simulink model "bldc_motor_sim_v2"  (R2024b)
settings: Solver=VariableStepAuto  StartTime=0.0  StopTime=1  RelTol=1e-3
undefined symbols (not defined in the file): closed_loop, D_m, DiscIntNeverNeededParam, J_t, L_ss, lambda_m, P, r_s, R_vs, V_bus
libraries: spsMosfetLib x6, spsSeriesRLCBranchLib x4, spsVoltageMeasurementLib x3, spsControlledCurrentSourceLib x3, embmathops x1, spsPWMGeneratorDCDCLib x1, spsDCVoltageSourceLib x1, sps_lib x1
settings Model: Creator=Aether  LastModifiedBy=Aether

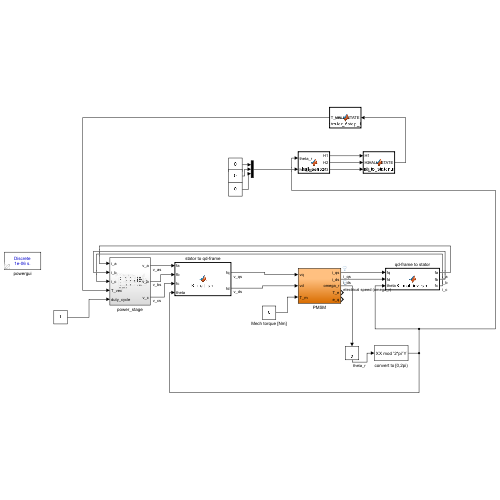
[thumbnail: Simulink's stored preview of the top-level diagram]
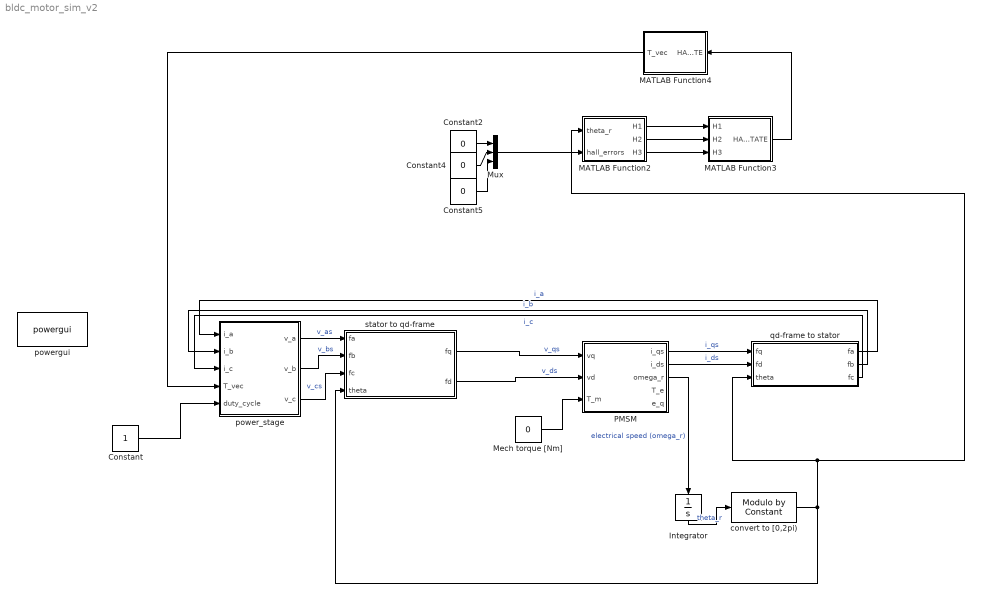
== system bldc_motor_sim_v2 ==
  Constant : Constant
  Constant2 : Constant  Value=0
  Constant4 : Constant  Value=0
  Constant5 : Constant  Value=0
  Integrator : Integrator
  MATLAB Function2 : MATLAB Function  TreatAsAtomicUnit=on
  MATLAB Function3 : MATLAB Function  TreatAsAtomicUnit=on
  MATLAB Function4 : MATLAB Function  TreatAsAtomicUnit=on
  Mech torque [Nm] : Constant  Value=0
  Mux : Mux  Inputs=3
  PMSM : Subsystem
  convert to [0,2pi) : embmathops/Modulo by Constant  Denominator=2*pi  SimulateUsing=Code generation
      settings: LibrarySourceBlock=embeddedMathLib/Modulo by Constant
  power_stage : Subsystem
  powergui : sps_lib/powergui  Priority=1  SimulationMode=Discrete  SampleTime=1e-6  frequency=60  Iterations=50  frequencyindice=0  Pbase=100e6  ErrMax=1e-4  UnitsV=kV  UnitsW=MW  buscounter=0  FunctionMessages=off  echomessages=off  EnableUseOfTLC=off  CurrentSourceSwitches=off  DisableSnubberDevices=off  DisableRonSwitches=off  DisableVfSwitches=off  DisplayEquations=off  AutomaticDiscreteSolvers=off  SolverType=Tustin/Backward Euler (TBE)  Interpol=off  ExternalGateDelay=off  methode=off  Ts=100  x0status=blocks  SPID=on  SwTol=0  HookPort=off  NonlinearTolerance=1e-4  nMaxIteration=100  ContinueOnMaxIteration=off  RestoreLinks=warning  ResistiveCurrentMeasurement=off  Frange=[0:2:500]  Ylog=off  Xlog=on  ShowGrid=off  save=off  variable=ZData  structure=0  ZoomFFT=off  StartTime=0.0  cycles=1  DisplayStyle=1  fundamental=60  FreqAxis=off  MaxFrequency=1000  frequencyindicesteady=1  RmsSteady=1  display=off
  qd-frame to stator : MATLAB Function  TreatAsAtomicUnit=on
  stator to qd-frame : MATLAB Function  TreatAsAtomicUnit=on
  wires:
  MATLAB Function4/1(T_vec) -> power_stage/4(T_vec)
  MATLAB Function2/2(H2) -> MATLAB Function3/2(H2)
  MATLAB Function2/3(H3) -> MATLAB Function3/3(H3)
  MATLAB Function3/1(HALL_STATE) -> MATLAB Function4/1(HALL_STATE)
  MATLAB Function2/1(H1) -> MATLAB Function3/1(H1)
  power_stage/1(v_a) -> stator to qd-frame/1(fa)  "v_as"
  power_stage/2(v_b) -> stator to qd-frame/2(fb)  "v_bs"
  power_stage/3(v_c) -> stator to qd-frame/3(fc)  "v_cs"
  stator to qd-frame/1(fq) -> PMSM/1(vq)  "v_qs"
  stator to qd-frame/2(fd) -> PMSM/2(vd)  "v_ds"
  Mech torque [Nm]/1 -> PMSM/3(T_m)
  PMSM/1(i_qs) -> qd-frame to stator/1(fq)  "i_qs"
  PMSM/2(i_ds) -> qd-frame to stator/2(fd)  "i_ds"
  Integrator/1 -> convert to [0,2pi)/1  "theta_r"
  PMSM/3(omega_r) -> Integrator/1  "electrical speed (omega_r)"
  convert to [0,2pi)/1 -> MATLAB Function2/1(theta_r), qd-frame to stator/3(theta), stator to qd-frame/4(theta)
  qd-frame to stator/1(fa) -> power_stage/1(i_a)  "i_a"
  qd-frame to stator/2(fb) -> power_stage/2(i_b)  "i_b"
  qd-frame to stator/3(fc) -> power_stage/3(i_c)  "i_c"
  Constant/1 -> power_stage/5(duty_cycle)
  Constant2/1 -> Mux/1
  Constant5/1 -> Mux/3
  Mux/1 -> MATLAB Function2/2(hall_errors)
  Constant4/1 -> Mux/2

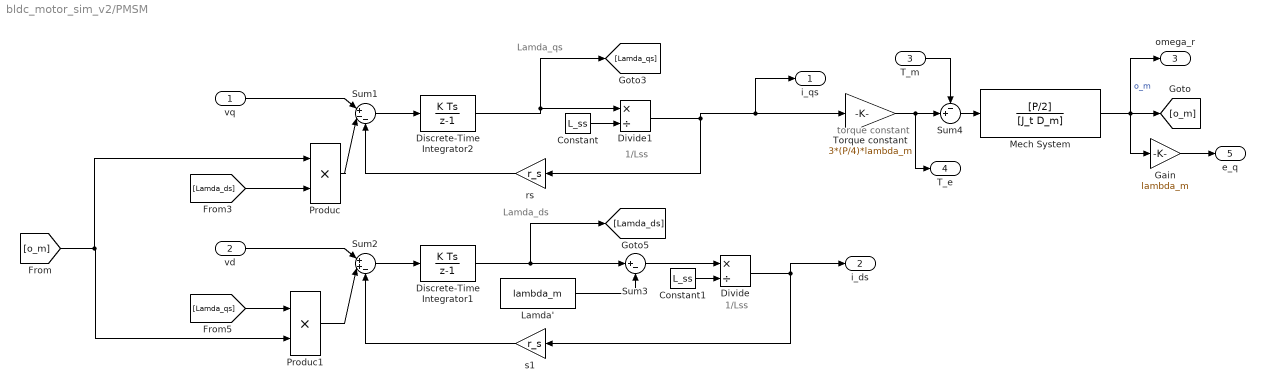
== system bldc_motor_sim_v2/PMSM ==
  note: torque constant
  note: Lamda_ds
  note: Lamda_qs
  note: 1/Lss
  note: 1/Lss
  vq : Inport
  vd : Inport  Port=2
  T_m : Inport  Port=3
  Constant : Constant  Value=L_ss
  Constant1 : Constant  Value=L_ss
  Discrete-Time Integrator1 : DiscreteIntegrator  SampleTime=-1  ICPrevOutput=DiscIntNeverNeededParam  ICPrevScaledInput=DiscIntNeverNeededParam
  Discrete-Time Integrator2 : DiscreteIntegrator  SampleTime=-1  ICPrevOutput=DiscIntNeverNeededParam  ICPrevScaledInput=DiscIntNeverNeededParam
  Divide : Product  Inputs=*/
  Divide1 : Product  Inputs=*/
  Gain : Gain  Gain=lambda_m
  Lamda' : Constant  Value=lambda_m
  Mech System : TransferFcn  Numerator=[P/2]  Denominator=[J_t D_m]
  Produc : Product  RndMeth=Zero
  Produc1 : Product  RndMeth=Zero
  Sum1 : Sum  Inputs=|+--
  Sum2 : Sum  Inputs=|++-
  Sum3 : Sum  Inputs=|+-
  Sum4 : Sum  Inputs=-+|
  Torque constant : Gain  Gain=3*(P/4)*lambda_m
  rs : Gain  Gain=r_s
  s1 : Gain  Gain=r_s
  i_qs : Outport
  i_ds : Outport  Port=2
  omega_r : Outport  Port=3
  T_e : Outport  Port=4
  e_q : Outport  Port=5
  wires:
  vd/1 -> Sum2/1
  vq/1 -> Sum1/1
  [Lamda_qs] -> Produc1/1
  [Lamda_ds] -> Produc/2
  [o_m] -> Produc1/2, Produc/1
  Lamda'/1 -> Sum3/2
  Sum3/1 -> Divide/1
  s1/1 -> Sum2/3
  Discrete-Time Integrator1/1 -> [Lamda_ds], Sum3/1
  Sum2/1 -> Discrete-Time Integrator1/1
  Produc1/1 -> Sum2/2
  Divide1/1 -> i_qs/1, Torque constant/1, rs/1
  rs/1 -> Sum1/3
  Discrete-Time Integrator2/1 -> [Lamda_qs], Divide1/1
  Sum1/1 -> Discrete-Time Integrator2/1
  Produc/1 -> Sum1/2
  Torque constant/1 -> Sum4/2, T_e/1
  Divide/1 -> i_ds/1, s1/1
  T_m/1 -> Sum4/1
  Sum4/1 -> Mech System/1
  Constant/1 -> Divide1/2
  Constant1/1 -> Divide/2
  Mech System/1 -> Gain/1, omega_r/1, [o_m]  "o_m"
  Gain/1 -> e_q/1

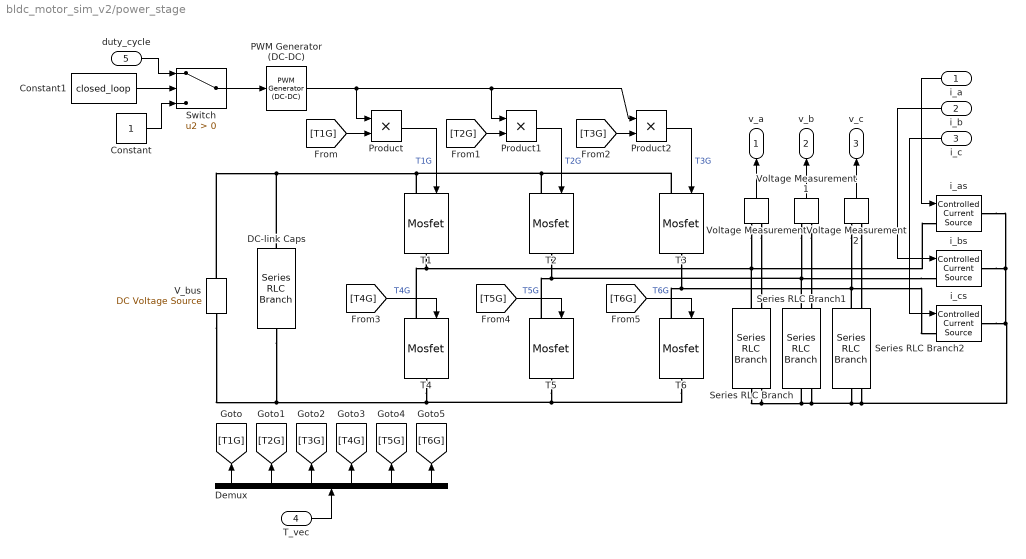
== system bldc_motor_sim_v2/power_stage ==
  i_a : Inport
  i_b : Inport  Port=2
  i_c : Inport  Port=3
  T_vec : Inport  Port=4
  duty_cycle : Inport  Port=5
  Constant : Constant
  Constant1 : Constant  Value=closed_loop
  DC-link Caps : spsSeriesRLCBranchLib/Series RLC Branch  LConnTagsString=__new0  RConnTagsString=__new0  BranchType=RC  Resistance=1e-6  Inductance=0  SetiL0=off  InitialCurrent=0  Capacitance=100e-6  Setx0=off  InitialVoltage=0  Measurements=None
  Demux : Demux  Outputs=6
  PWM Generator (DC-DC) : spsPWMGeneratorDCDCLib/PWM Generator (DC-DC)  Fsw=f_SW_Hz  Ts=0
  Product : Product
  Product1 : Product
  Product2 : Product
  Series RLC Branch : spsSeriesRLCBranchLib/Series RLC Branch  LConnTagsString=__new0  RConnTagsString=__new0  BranchType=R  Resistance=R_vs  Inductance=0  SetiL0=off  InitialCurrent=0  Capacitance=inf  Setx0=off  InitialVoltage=0  Measurements=None
  Series RLC Branch1 : spsSeriesRLCBranchLib/Series RLC Branch  LConnTagsString=__new0  RConnTagsString=__new0  BranchType=R  Resistance=R_vs  Inductance=0  SetiL0=off  InitialCurrent=0  Capacitance=inf  Setx0=off  InitialVoltage=0  Measurements=None
  Series RLC Branch2 : spsSeriesRLCBranchLib/Series RLC Branch  LConnTagsString=__new0  RConnTagsString=__new0  BranchType=R  Resistance=R_vs  Inductance=0  SetiL0=off  InitialCurrent=0  Capacitance=inf  Setx0=off  InitialVoltage=0  Measurements=None
  Switch : Switch  Criteria=u2 > Threshold  SaturateOnIntegerOverflow=off  InputSameDT=off
  T{1..6} (6 alike) : spsMosfetLib/Mosfet  Ron=R_dsON_Ohm  Lon=0  Rd=0.01  Vfd=0.7  IC=0  Rs=1e5  Cs=inf  Measurements=off
  V_bus : spsDCVoltageSourceLib/DC Voltage Source  Amplitude=V_bus  Measurements=None
  Voltage Measurement : spsVoltageMeasurementLib/Voltage Measurement  PhasorSimulation=off  OutputType=Complex  PSBequivalent=0
  Voltage Measurement1 : spsVoltageMeasurementLib/Voltage Measurement  PhasorSimulation=off  OutputType=Complex  PSBequivalent=0
  Voltage Measurement2 : spsVoltageMeasurementLib/Voltage Measurement  PhasorSimulation=off  OutputType=Complex  PSBequivalent=0
  i_as : spsControlledCurrentSourceLib/Controlled Current Source  Initialize=on  Source_Type=AC  Amplitude=0  Phase=0  Frequency=0  Measurements=None
  i_bs : spsControlledCurrentSourceLib/Controlled Current Source  Initialize=on  Source_Type=AC  Amplitude=0  Phase=0  Frequency=0  Measurements=None
  i_cs : spsControlledCurrentSourceLib/Controlled Current Source  Initialize=on  Source_Type=AC  Amplitude=0  Phase=0  Frequency=0  Measurements=None
  v_a : Outport
  v_b : Outport  Port=2
  v_c : Outport  Port=3
  wires:
  T_vec/1 -> Demux/1
  Product1/1 -> T2/1  "T2G"
  PWM Generator (DC-DC)/1 -> Product/1, Product2/1, Product1/1
  Demux/6 -> [T6G]
  [T4G] -> T4/1  "T4G"
  [T5G] -> T5/1  "T5G"
  Demux/4 -> [T4G]
  Voltage Measurement/1 -> v_a/1
  [T2G] -> Product1/2
  Voltage Measurement1/1 -> v_b/1
  Voltage Measurement2/1 -> v_c/1
  i_a/1 -> i_as/1
  Demux/1 -> [T1G]
  Demux/5 -> [T5G]
  [T6G] -> T6/1  "T6G"
  i_c/1 -> i_cs/1
  Product/1 -> T1/1  "T1G"
  [T3G] -> Product2/2
  i_b/1 -> i_bs/1
  Product2/1 -> T3/1  "T3G"
  Demux/2 -> [T2G]
  Demux/3 -> [T3G]
  [T1G] -> Product/2
  duty_cycle/1 -> Switch/1
  Constant/1 -> Switch/3
  Constant1/1 -> Switch/2
  Switch/1 -> PWM Generator (DC-DC)/1
  connections:
  i_bs/LConn1 -- Voltage Measurement1/LConn1 -- Series RLC Branch1/LConn1 -- T2/RConn1 -- T5/LConn1
  DC-link Caps/RConn1 -- V_bus/LConn1 -- T4/RConn1 -- T6/RConn1 -- T5/RConn1
  DC-link Caps/LConn1 -- V_bus/RConn1 -- T1/LConn1 -- T3/LConn1 -- T2/LConn1
  T4/LConn1 -- T1/RConn1 -- Voltage Measurement/LConn1 -- Series RLC Branch/LConn1 -- i_as/LConn1
  T3/RConn1 -- T6/LConn1 -- Voltage Measurement2/LConn1 -- Series RLC Branch2/LConn1 -- i_cs/LConn1
  Series RLC Branch/RConn1 -- Voltage Measurement/LConn2 -- i_bs/RConn1 -- i_as/RConn1 -- i_cs/RConn1 -- Voltage Measurement2/LConn2 -- Series RLC Branch2/RConn1 -- Voltage Measurement1/LConn2 -- Series RLC Branch1/RConn1

== matlab function bldc_motor_sim_v2/qd-frame to stator ==
  data: fa output; fb output; fc output; fq input; fd input; theta input
function [fa,fb,fc] = K_mat_inv_sim(fq,fd,theta)
[fa,fb,fc] = K_mat_inv(fq,fd,theta);

== matlab function bldc_motor_sim_v2/stator to qd-frame ==
  data: fa input; fq output; fb input; fc input; theta input; fd output
function [fq,fd] = K_mat_sim(fa,fb,fc,theta)
[fq,fd] = K_mat(fa,fb,fc,theta);

== matlab function bldc_motor_sim_v2/MATLAB Function2 ==
  data: theta_r input; H1 output; hall_errors input; H2 output; H3 output
function [H1,H2,H3] = hall_sensor(theta_r, hall_errors)
%HALL_SENSOR Obtain hall signals from electrical angle
%   Detailed explanation goes here
H1 = 0;
H2 = 0;
H3 = 0;
theta_r1 = mod(theta_r - hall_errors(1), 2*pi);
theta_r2 = mod(theta_r - hall_errors(2), 2*pi);
theta_r3 = mod(theta_r - hall_errors(3), 2*pi);

if ((0 <= theta_r1 && theta_r1 <= pi/2) || (3*pi/2 <= theta_r1 &&  theta_r1 <=2*pi))
    H1 = 1;
end
if (pi/6 <= theta_r2 && theta_r2 <=7*pi/6)
    H2 = 1;
end
if (5*pi/6 <= theta_r3 && theta_r3 <=11*pi/6)
    H3 = 1;
end
end

== matlab function bldc_motor_sim_v2/MATLAB Function3 ==
  data: H1 input; HALL_STATE output; H2 input; H3 input
function HALL_STATE = hall_to_statenum(H1,H2,H3)
HALL_STATE = 4*H1 + 2*H2 + H3;

== matlab function bldc_motor_sim_v2/MATLAB Function4 ==
  data: HALL_STATE input; T_vec output
function T_vec = controller_6step_120(HALL_STATE)
%CONTROLLER_6STEP_180 Summary of this function goes here
%   Detailed explanation goes here

T_vec = zeros(6,1);
% HALL_STATE = 4*H1 + 2*H2 + H3;
if (HALL_STATE > 6)
    fprintf("Hall = %.3f", HALL_STATE)
    error("Invalid hall state!!")
end

switch HALL_STATE
    case 4 % State I
        T_vec([1,5]) = 1;
    case 6 % State II
        T_vec([1,6]) = 1;
    case 2 % State III
        T_vec([2,6]) = 1;
    case 3 % State IV
        T_vec([2,4]) = 1;
    case 1 % State V
        T_vec([3,4]) = 1;
    case 5 % State VI
        T_vec([3,5]) = 1;
    otherwise
end
end
